simulink model "p7"  (R2020a)
settings: Solver=VariableStepAuto  StartTime=0.0  StopTime=3  RelTol=1e-3
settings Model: Creator=a.kochnov  LastModifiedBy=a.kochnov

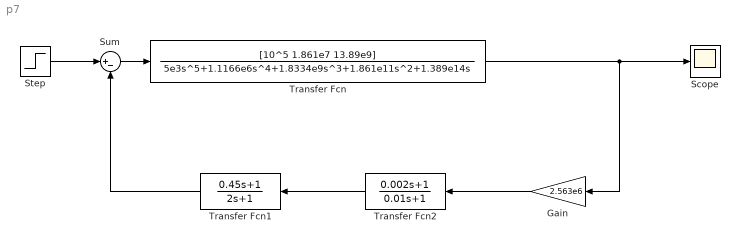
== system p7 ==
  Gain : Gain  Gain=2.563e6
  Scope : Scope
  Step : Step  SampleTime=0
  Sum : Sum  Inputs=|+-
  Transfer Fcn : TransferFcn  Numerator=[10^5 1.861e7 13.89e9]  Denominator=[5e3 1.1166e6 1.8334e9 1.861e11 1.389e14 0]
  Transfer Fcn1 : TransferFcn  Numerator=[0.45 1]  Denominator=[2 1]
  Transfer Fcn2 : TransferFcn  Numerator=[0.002 1]  Denominator=[0.01 1]
  wires:
  Transfer Fcn/1 -> Gain/1, Scope/1
  Gain/1 -> Transfer Fcn2/1
  Transfer Fcn2/1 -> Transfer Fcn1/1
  Transfer Fcn1/1 -> Sum/2
  Sum/1 -> Transfer Fcn/1
  Step/1 -> Sum/1
